simulink model "simulink_L2narma"  (R2018a)
settings: Solver=FixedStepDiscrete  StartTime=0.0  StopTime=1000  FixedStep=1  RelTol=1e-3
libraries: neural x1
settings Model: Creator=Labit  LastModifiedBy=vladi

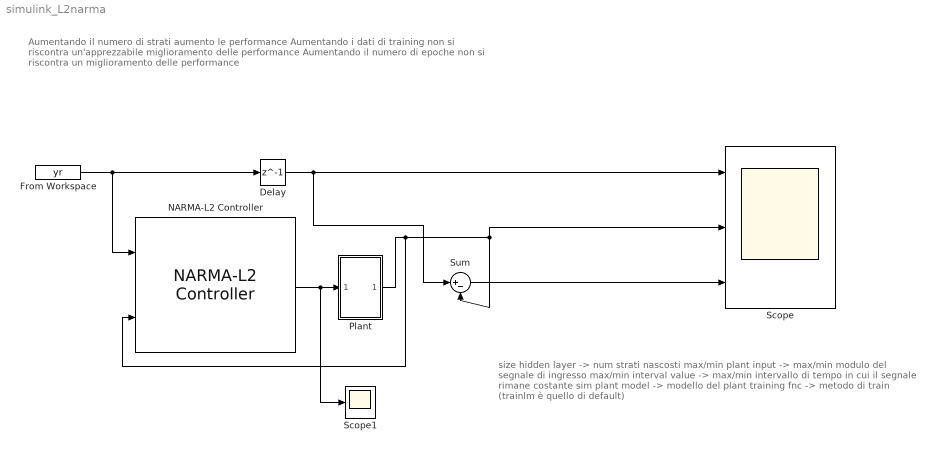
== system simulink_L2narma ==
  note: Aumentando il numero di strati aumento le performance
      | Aumentando i dati di training non si riscontra un'apprezzabile miglioramento delle performance
      | Aumentando il numero di epoche non si riscontra un miglioramento delle performance
  note: size hidden layer -> num strati nascosti
      | max/min plant input -> max/min modulo del segnale di ingresso
      | max/min interval value -> max/min intervallo di tempo in cui il segnale rimane costante
      | sim plant model -> modello del plant
      | training fnc -> metodo di train (trainlm è quello di default)
  Delay : Delay  DelayLength=1
  From Workspace : FromWorkspace  VariableName=yr  SampleTime=0
  NARMA-L2 Controller : neural/Control Systems/NARMA-L2 Controller  Normalize=0  IW1_1=[3.8139668417404157807;3.8815259750513657622;-3.2748939026658394624;-3.9053410376066932663;-3.9918911414699991269;3.9617695367724268252;3.7625515611634710034;3.4792158481124775271;-4.494892344131133477;-3.630501821281530983]  IW3_2=[3.107722634884295676;-3.63539395822912903;4.1347479444800159243;1.4466577122526385057;3.9194109340407985442;4.0902183452004265973;-3.3334755696126863178;4.7709785865149694217;3.7531539358472731926;-3.381309825628808774]  IW5_3=1.2119482686227274204  LW2_1=[0.21333823344687477541 -0.0070406795523092592995 -0.47496850922246669491 -2.0134951659314324068 1.7145644906181398692 -2.3087048236045868421 0.71499464688394964718 0.58652276660688851262 -0.29512503808507628555 0.018432258193309937477]  LW4_3=[-1.1063469404212664671 -0.099450486535374360564 0.95617524382472052213 -0.46143587615251924205 -1.0335709352472535194 0.27950775340473149599 -2.5854008364531435582 -2.7160008399382067346 -0.015655045047843148959 -1.3492927486196748532]  LW5_4=-1.2401094516026132109  LW6_5=-1.2985360848145661716  LW6_2=-0.18012219517028660309  B1=[-14.030894086278026478;-10.904217013967640426;8.0978085963681856185;5.1004539200099916485;1.4117176266810222973;1.5223818948248493133;4.9488930905456030018;8.0309642541310939379;-10.633295353449755183;-14.078725637009846139]  B2=0.66890276405500292967  B3=[-14.236624680391679831;10.988192337402621135;-7.8935896132525043001;-6.3539009784577276108;-1.5349211517952128236;1.154754031930957936;-5.0587916083739052908;8.3781029258292090134;10.936398782319368905;-14.148438906026942874]  B4=1.0789266477707291081  Limit_output=1  min_output=-1.6  max_output=1.6  Use_Previous_Weights=1  Ts=1  S1=10  Ni=1  Nj=1  sim_file=simulink_L2  trainfun=trainlm  Use_validation=1  Use_Testing=1  max_i=0.6  min_i=-0.6  max_i_int=20  min_i_int=1  sam_training=1500  epochs=200  minp=-0.59823129250737361318  maxp=0.59811034980767641134  mint=-4.3520705222512647836  maxt=0.59811034980767641134
      settings: SourceProductName=Neural Network Toolbox  SourceProductBaseCode=NN
  "Plant " : Subsystem
  Scope : Scope  NumInputPorts=3
  Scope1 : Scope
  Sum : Sum  Inputs=|+-
  wires:
  "Plant "/1(y(k)) -> NARMA-L2 Controller/2, Sum/2, Scope/2
  NARMA-L2 Controller/1 -> Scope1/1, "Plant "/1(u(k))
  From Workspace/1 -> NARMA-L2 Controller/1, Delay/1
  Delay/1 -> Sum/1, Scope/1
  Sum/1 -> Scope/3

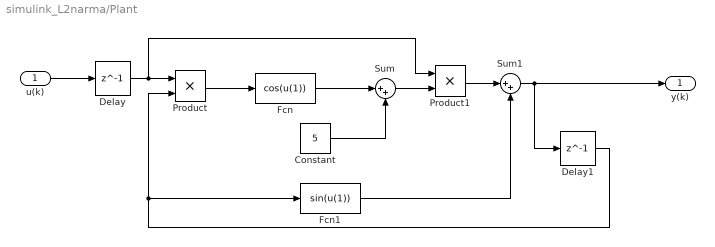
== system simulink_L2narma/Plant  ==
  u(k) : Inport
  Constant : Constant  Value=5
  Delay : Delay  DelayLength=1  InitialCondition=0
  Delay1 : Delay  DelayLength=1  InitialCondition=0
  Fcn : Fcn  Expr=cos(u(1))
  Fcn1 : Fcn  Expr=sin(u(1))
  Product : Product
  Product1 : Product
  Sum : Sum  Inputs=|++
  Sum1 : Sum  Inputs=|++
  y(k) : Outport
  wires:
  Delay/1 -> Product1/1, Product/1
  Delay1/1 -> Fcn1/1, Product/2
  Product1/1 -> Sum1/1
  Fcn/1 -> Sum/1
  Fcn1/1 -> Sum1/2
  Sum1/1 -> y(k)/1, Delay1/1
  Sum/1 -> Product1/2
  Product/1 -> Fcn/1
  Constant/1 -> Sum/2
  u(k)/1 -> Delay/1
